simulink model "NewMODEL"  (R2023a)
settings: Solver=VariableStepAuto  StartTime=0.0  StopTime=6  RelTol=1e-3
values from neighbouring files (symbols this model uses):
  A_lift = 3    [Main.m]    (also in SweepTest.m; myActiveSuspensions.mat)
  AO = A-KO*C    [Main.m]    (also in SweepTest.m; myActiveSuspensions.mat = [-6.29015203402 -9209.07677924 -1030.51480744 -503585.757509)
  Ap = 3.35e-4    (= 0.000335)    [Main.m]    (also in SweepTest.m; myActiveSuspensions.mat)
  BO = B1-KO*D1    [Main.m]    (also in SweepTest.m; myActiveSuspensions.mat = [0 0 0 0 154.5])
  Cd_lift = 0.5    [Main.m]    (also in SweepTest.m; myActiveSuspensions.mat)
  Ceps = [1 0 0 0 0 0 ... (first row only)    [Main.m]    (also in SweepTest.m; myActiveSuspensions.mat = [1 0 0 0 0 0 -98.3050847458 1 0 1 0 0 ... (48 elements, 8x6))
  D1eps = [0; 0; 0; 0; 0; 0; 0; 0]    [Main.m]    (also in SweepTest.m; myActiveSuspensions.mat = [0 0 0 0 0 0 0 0])
  DT = 1e-4    (= 0.0001)    [Main.m]    (also in SweepTest.m; myActiveSuspensions.mat)
  e0 = y0(1) - r0    [Main.m]    (also in SweepTest.m; myActiveSuspensions.mat = 0)
  KI = K(:,n+1:n+m)    [Main.m]    (also in SweepTest.m; myActiveSuspensions.mat = -0.35355339059)
  KO = Km.'    [Main.m]    (also in SweepTest.m; myActiveSuspensions.mat = [0.176588896426 58.0307081185 2.94746555023 -226.466108515 -)
  KS = K(:,1:n)    [Main.m]    (also in SweepTest.m; myActiveSuspensions.mat = [3465.7518789 327.330365312 55.983697187 9.36087983472 -400.)
  mi = 1e-7    (= 1e-07)    [Main.m]    (also in SweepTest.m; myActiveSuspensions.mat)
  myVars = rmfield(myVars, "kerO")    [Main.m]    (also in SweepTest.m = rmfield(myVars, "mdl"))
  n = size(V)    [JCF.m]    (also in Main.m = 5; SweepTest.m = 5; myActiveSuspensions.mat = 5)
  p = 1    [Main.m]    (also in SweepTest.m; myActiveSuspensions.mat)
  q = length(index{i})    [JCF.m]    (also in Main.m = 3; SweepTest.m = 3; myActiveSuspensions.mat = 3)
  r0 = - g*ms/ks + l0s + Lift/ks    (= 0.597040517241)    [Main.m]    (also in SweepTest.m; myActiveSuspensions.mat)
  rho_lift = 1.225    [Main.m]    (also in SweepTest.m; myActiveSuspensions.mat)
  v = 10    [Main.m]    (also in SweepTest.m; myActiveSuspensions.mat)
  w0 = [d0; nu0; r0]    [Main.m]    (also in SweepTest.m; myActiveSuspensions.mat = [0 -91.875 0 0 0 0.597040517241])
  x0 = [- g*ms/ks + l0s + Lift/ks ... (first row only)    [Main.m]    (also in SweepTest.m; myActiveSuspensions.mat = [0.597040517241 0 0.3385371843 0 0])
  x_init = [(- g*ms/ks + l0s + Lift/ks) - Diseq ... (first row only)    [Main.m]    (also in SweepTest.m; myActiveSuspensions.mat = [0.597040517241 0 0.3385371843 0 0])
  x_tilde_init = x_init - x0    [Main.m]    (also in SweepTest.m; myActiveSuspensions.mat = [0 0 0 0 0])
  XOinit = x_tilde_init    [Main.m]    (also in SweepTest.m; myActiveSuspensions.mat = [0 0 0 0 0])
  y0 = [x0(1) ... (first row only)    [Main.m]    (also in SweepTest.m; myActiveSuspensions.mat = [0.597040517241 0.935577701542 6.16606577473e-15])
libraries: simulink x3
settings Model: Creator=aleze  LastModifiedBy=aleze

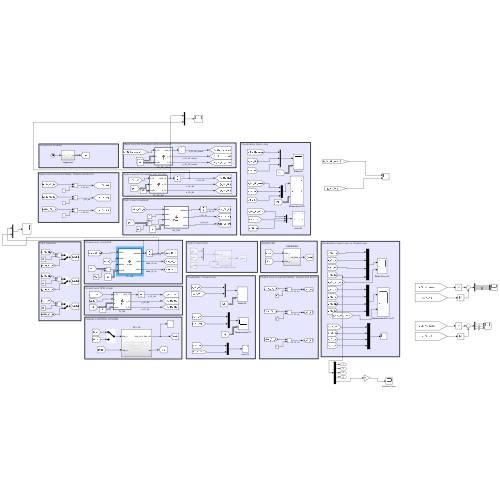
[thumbnail: Simulink's stored preview of the top-level diagram]
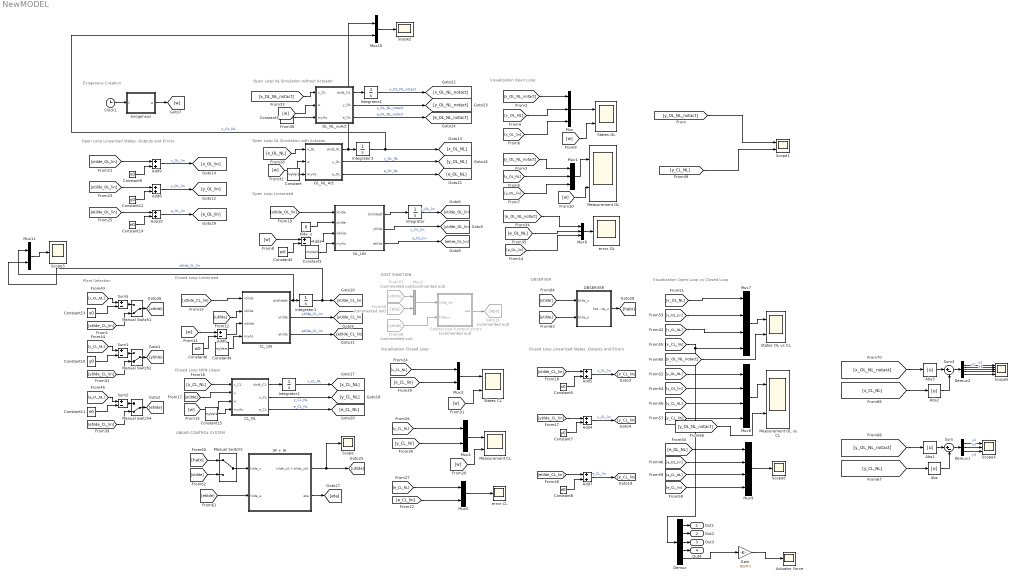
== system NewMODEL ==
  note: Closed Loop Linearized
  note: Open Loop NL Simulation without Actuator
  note: Closed Loop NON Linear
  note: Open Loop Linearized
  note: Exogenous Creation
  note: LINEAR CONTROL SYSTEM
  note: Visualization Open Loop
  note: OBSERVER
  note: Visualization Closed Loop
  note: Open Loop Linearized States, Outputs and Errors
  note: Visualization Open Loop vs Closed Loop
  note: Plant Selection
  note: Closed Loop Linearized States, Outputs and Errors
  note: Open Loop NL Simulation with Actuator
  note: COST FUNCTION
  Abs{,1..3} (4 alike) : Abs  SaturateOnIntegerOverflow=off
  Actuator Force : Scope
  Add{4..5,7..10} (6 alike) : Sum
  Add2 : Sum  Inputs=+-
  Add6 : Sum  Inputs=+-
  CL_LIN : MATLAB Function  TreatAsAtomicUnit=on
  CL_NL : MATLAB Function  TreatAsAtomicUnit=on
  Clock1 : Clock
  Constant{,1,3..4,15} (5 alike) : Constant  Value=myVars  OutDataTypeStr=Bus: slBus1
  Constant10 : Constant  Value=y0
  Constant11 : Constant  Value=e0
  Constant12 : Constant  Value=y0
  Constant13 : Constant  Value=x0
  Constant14 : Constant  Value=e0
  Constant2 : Constant  Value=w0
  Constant5 : Constant  Value=x0
  Constant6 : Constant  Value=w0
  Constant7 : Constant  Value=y0
  Constant8 : Constant  Value=e0
  Constant9 : Constant  Value=x0
  Control cost function errors : Subsystem  Commented=on
  Demux : Demux  Outputs=5
  Demux1 : Demux  Outputs=3
  Demux2 : Demux  Outputs=5
  From37 : From  Commented=on  GotoTag=xtilde
  From38 : From  Commented=on  GotoTag=utilde
  From40 : From  Commented=on  GotoTag=eta
  Gain : Gain  Gain=Ap/mi
  Goto15 : Goto  Commented=on  GotoTag=eps
  Integrator : Integrator  InitialCondition=x_tilde_init
  Integrator1 : Integrator  InitialCondition=x_tilde_init
  Integrator2 : Integrator  InitialCondition=x_init
  Integrator3 : Integrator  InitialCondition=x_init
  Integrator4 : Integrator  InitialCondition=x_init
  Manual Switch1 : ManualSwitch  CurrentSetting=0
  Manual Switch2 : ManualSwitch  CurrentSetting=0
  Manual Switch4 : ManualSwitch  CurrentSetting=0
  Manual Switch5 : ManualSwitch
  Measurement CL : Scope  NumInputPorts=2
  Measurement OL : Scope  NumInputPorts=2
  Measurement OL vs CL : Scope  NumInputPorts=2
  Mux : Mux  Inputs=3
  Mux1 : Mux  Inputs=3
  Mux{3..5,10..11} (5 alike) : Mux  Inputs=2
  Mux2 : Mux  Commented=on  Inputs=2
  Mux6 : Mux  Inputs=3
  Mux7 : Mux
  Mux8 : Mux
  Mux9 : Mux
  OBSERVER : Subsystem
  OL_LIN : MATLAB Function  TreatAsAtomicUnit=on
  OL_NL_Act : MATLAB Function  TreatAsAtomicUnit=on
  OL_NL_noAct : MATLAB Function  TreatAsAtomicUnit=on
  SF + IA : Subsystem
  Scope{,2..3,6} (4 alike) : Scope
  Scope1 : Scope  NumInputPorts=2
  Scope4 : Scope  NumInputPorts=3
  Scope5 : Scope  NumInputPorts=5
  States CL : Scope  NumInputPorts=2
  States OL : Scope  NumInputPorts=2
  States OL vs CL : Scope  NumInputPorts=2
  Sum : Sum  Inputs=|+-
  Sum1 : Sum  Inputs=+-
  Sum2 : Sum  Inputs=+-
  Sum3 : Sum  Inputs=|+-
  Sum5 : Sum  Inputs=+-
  error CL : Scope
  error OL : Scope
  exogenous : Subsystem
  tilde_u : Constant  Value=0  VectorParams1D=off
  Out1 : Outport
  Out2 : Outport  Port=2
  Out3 : Outport  Port=3
  Out4 : Outport  Port=4
  wires:
  [xtilde_CL_lin] -> CL_LIN/1(xtilde)
  [x_OL_NL] -> OL_NL_Act/1(x_OL)
  Sum5/1 -> Manual Switch1/1
  [xtilde_CL_lin] -> Manual Switch1/2
  Mux6/1 -> error OL/1
  Add7/1 -> [e_CL_lin]  "e_CL_lin"
  Add5/1 -> [x_CL_lin]  "x_CL_lin"
  Demux1/3 -> Scope4/3  "y3"
  [x_OL_NL_notact] -> OL_NL_noAct/1(x_OL)
  Integrator2/1 -> [x_CL_NL]  "x_CL_NL"
  Constant10/1 -> Sum1/2
  [x_CL_NL] -> Abs2/1
  [utilde] -> CL_LIN/2(utilde)
  OL_NL_Act/3(e_OL) -> [e_OL_NL]  "e_OL_NL"
  Constant6/1 -> Add6/2
  [w] -> Add6/1
  [x_CL_lin] -> Mux3/2
  Sum2/1 -> Manual Switch4/1
  [x_CL_NL] -> Mux7/3
  [w] -> States OL/2
  [y_OL_NL_notact] -> Scope1/1
  OL_LIN/1(dxtildedt) -> Integrator/1
  Clock1/1 -> exogenous/1(t)
  [ytilde_CL_lin] -> Manual Switch2/2
  Integrator1/1 -> Mux11/2, [xtilde_CL_lin]  "xtilde_CL_lin"
  CL_NL/2(y_CL) -> [y_CL_NL]  "y_CL_NL"
  OL_NL_noAct/3(e_OL) -> [e_OL_NL_notact]  "e_OL_NL_notact"
  [w] -> Measurement CL/2
  [x_OL_NL] -> Mux7/1
  Manual Switch1/1 -> [xtilde]
  [y_CL_NL] -> Sum1/1
  OL_NL_Act/2(y_OL) -> [y_OL_NL]  "y_OL_NL"
  Manual Switch4/1 -> [etilde]
  [w] -> States CL/2
  Constant5/1 -> Add5/2
  [e_CL_NL] -> Mux9/3
  [x_OL_NL] -> Mux/2
  OL_NL_Act/1(dxdt_OL) -> Mux10/1, Integrator3/1
  [y_OL_NL] -> Mux1/2
  Control cost function errors/1(eps) -> Goto15/1
  Add2/1 -> OL_LIN/3(wtilde)
  Mux1/1 -> Measurement OL/1
  CL_NL/3(e_CL) -> [e_CL_NL]  "e_CL_NL"
  exogenous/1(w) -> [w]
  [x_CL_lin] -> Demux/1, Mux7/4
  Mux4/1 -> Measurement CL/1
  OL_NL_noAct/1(dxdt_OL) -> Integrator4/1
  Constant11/1 -> Sum2/2
  [w] -> Measurement OL/2
  Sum/1 -> Demux1/1
  [e_OL_NL] -> Mux6/2
  [e_OL_lin] -> Mux6/3
  CL_LIN/2(ytilde) -> [ytilde_CL_lin]  "ytilde_CL_lin"
  [etilde_OL_lin] -> Add10/1
  CL_LIN/1(dxtildedt) -> Mux11/1, Integrator1/1
  Abs/1 -> Sum/2
  Demux/2 -> Out2/1
  Demux/5 -> Gain/1
  Mux/1 -> States OL/1
  Mux11/1 -> Scope3/1
  [ytilde] -> OBSERVER/2(tilde_y)
  Demux1/2 -> Scope4/2  "y2"
  Gain/1 -> Actuator Force/1
  Mux10/1 -> Scope2/1
  From37/1 -> Mux2/1
  Demux2/3 -> Scope5/3  "y3"
  Demux2/1 -> Scope5/1  "y1"
  Add9/1 -> [x_OL_lin]  "x_OL_lin"
  [etilde_CL_lin] -> Manual Switch4/2
  Demux1/1 -> Scope4/1  "y1"
  Demux2/2 -> Scope5/2  "y2"
  Mux8/1 -> Measurement OL vs CL/1
  [w] -> OL_NL_Act/2(w)
  [y_CL_NL] -> Mux8/3
  [e_CL_lin] -> Mux5/2
  Abs2/1 -> Sum3/2
  Integrator/1 -> [xtilde_OL_lin]  "x_OL_lin"
  [x_CL_NL] -> CL_NL/1(x_CL)
  Mux5/1 -> error CL/1
  Mux9/1 -> Scope6/1
  Add10/1 -> [e_OL_lin]  "e_OL_lin"
  [x_OL_lin] -> Mux7/2
  [w] -> Add2/1
  Constant12/1 -> Add8/2
  [e_CL_lin] -> Mux9/4
  Sum1/1 -> Manual Switch2/1
  [ytilde_OL_lin] -> Add8/1
  CL_NL/1(dxdt_CL) -> Integrator2/1
  Mux3/1 -> States CL/1
  Constant14/1 -> Add10/2
  [e_CL_NL] -> Mux5/1
  [y_OL_NL] -> Mux8/1
  Mux7/1 -> States OL vs CL/1
  [e_OL_NL] -> Mux9/1
  [y_OL_lin] -> Mux8/2
  SF + IA/2(eta) -> [eta]
  Demux2/5 -> Scope5/5
  Abs1/1 -> Sum/1
  [x_OL_NL_notact] -> Mux/1
  OL_LIN/2(ytilde) -> [ytilde_OL_lin]  "y_OL_lin"
  [w] -> OL_NL_noAct/2(w)
  [utilde] -> CL_NL/2(u)
  Constant13/1 -> Sum5/2
  Mux2/1 -> Control cost function errors/1(tilde_xe)
  [y_OL_NL_notact] -> Abs1/1
  Constant/1 -> OL_NL_Act/3(myAs)
  [e_CL_NL] -> Sum2/1
  [utilde] -> OBSERVER/1(tilde_u)
  [y_CL_lin] -> Mux8/4
  Constant1/1 -> OL_LIN/4(myAs)
  Constant7/1 -> Add4/2
  Constant3/1 -> OL_NL_noAct/3(myAs)
  [w] -> CL_NL/3(w)
  Constant15/1 -> CL_NL/4(myAs)
  [y_CL_lin] -> Mux4/2
  Constant4/1 -> CL_LIN/4(myAs)
  [hatx] -> Manual Switch5/1
  [xtilde_OL_lin] -> OL_LIN/1(xtilde)
  Constant8/1 -> Add7/2
  Demux/4 -> Out4/1
  OL_LIN/3(etilde) -> [etilde_OL_lin]  "e_OL_lin"
  [x_CL_NL] -> Sum5/1
  Manual Switch5/1 -> SF + IA/1(tilde_x)
  [ytilde_CL_lin] -> Add4/1
  tilde_u/1 -> OL_LIN/2(utilde)
  [x_OL_NL_notact] -> Abs3/1
  [y_OL_NL_notact] -> Mux1/1
  [y_CL_NL] -> Scope1/2
  Add6/1 -> CL_LIN/3(wtilde)
  [etilde_CL_lin] -> Add7/1
  Demux/1 -> Out1/1
  From38/1 -> Control cost function errors/2(tilde_u)
  Demux2/4 -> Scope5/4
  Constant2/1 -> Add2/2
  SF + IA/1(tilde_uS + tilde_uIA) -> [utilde], Scope/1
  Abs3/1 -> Sum3/1
  [y_CL_NL] -> Mux4/1
  Integrator3/1 -> Mux10/2, [x_OL_NL]  "x_OL_NL"
  Manual Switch2/1 -> [ytilde]
  [e_OL_NL_notact] -> Mux6/1
  [xtilde_CL_lin] -> Add5/1
  [xtilde] -> Manual Switch5/2
  OBSERVER/1(hat_tilde_x) -> [hatx]
  Add4/1 -> [y_CL_lin]  "y_CL_lin"
  [y_OL_NL_notact] -> Measurement OL vs CL/2
  CL_LIN/3(etilde) -> [etilde_CL_lin]  "etilde_CL_lin"
  Demux/3 -> Out3/1
  [etilde] -> SF + IA/2(tilde_e)
  [e_OL_lin] -> Mux9/2
  [y_OL_lin] -> Mux1/3
  [x_CL_NL] -> Mux3/1
  Integrator4/1 -> [x_OL_NL_notact]  "x_OL_NL_notact"
  [x_OL_NL_notact] -> States OL vs CL/2
  [y_CL_NL] -> Abs/1
  From40/1 -> Mux2/2
  OL_NL_noAct/2(y_OL) -> [y_OL_NL_notact]  "y_OL_NL_notact"
  [xtilde_OL_lin] -> Add9/1
  Constant9/1 -> Add9/2
  Add8/1 -> [y_OL_lin]  "y_OL_lin"
  [x_OL_lin] -> Mux/3
  Sum3/1 -> Demux2/1

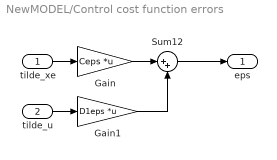
== system NewMODEL/Control cost function errors ==
  tilde_xe : Inport
  tilde_u : Inport  Port=2
  Gain : Gain  Gain=Ceps  Multiplication=Matrix(K*u)
  Gain1 : Gain  Gain=D1eps  Multiplication=Matrix(K*u)
  Sum12 : Sum  Inputs=|++
  eps : Outport
  wires:
  Gain1/1 -> Sum12/2
  Gain/1 -> Sum12/1
  Sum12/1 -> eps/1
  tilde_xe/1 -> Gain/1
  tilde_u/1 -> Gain1/1

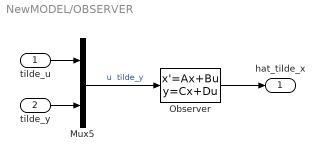
== system NewMODEL/OBSERVER ==
  tilde_u : Inport
  tilde_y : Inport  Port=2
  Mux5 : Mux  Inputs=2
  Observer : StateSpace  A=AO  B=[BO KO]  C=eye(n)  D=zeros(n, p+q)  InitialCondition=XOinit  ParameterTunability=Unconstrained
  hat_tilde_x : Outport
  wires:
  tilde_u/1 -> Mux5/1
  tilde_y/1 -> Mux5/2
  Mux5/1 -> Observer/1  "u  tilde_y"
  Observer/1 -> hat_tilde_x/1

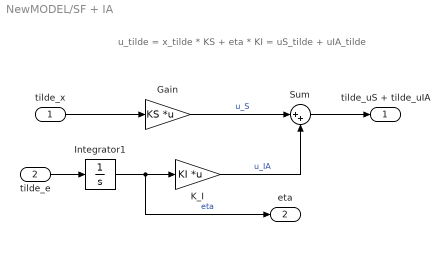
== system NewMODEL/SF + IA ==
  note: u_tilde = x_tilde * KS + eta * KI = uS_tilde + uIA_tilde
  tilde_x : Inport
  tilde_e : Inport  Port=2
  Gain : Gain  Gain=KS  Multiplication=Matrix(K*u)
  Integrator1 : Integrator
  K_I : Gain  Gain=KI  Multiplication=Matrix(K*u)
  Sum : Sum  Inputs=|++
  tilde_uS + tilde_uIA : Outport
  eta : Outport  Port=2
  wires:
  Integrator1/1 -> eta/1, K_I/1  "eta"
  tilde_e/1 -> Integrator1/1
  tilde_x/1 -> Gain/1
  K_I/1 -> Sum/2  "u_IA"
  Sum/1 -> tilde_uS + tilde_uIA/1
  Gain/1 -> Sum/1  "u_S"

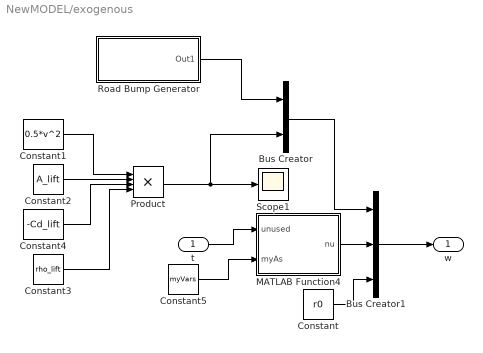
== system NewMODEL/exogenous ==
  t : Inport
  Bus Creator : BusCreator  Inputs=2
  Bus Creator1 : BusCreator  Inputs=3
  Constant : Constant  Value=r0
  Constant1 : Constant  Value=0.5*v^2  SampleTime=DT
  Constant2 : Constant  Value=A_lift  SampleTime=DT
  Constant3 : Constant  Value=rho_lift  SampleTime=DT
  Constant4 : Constant  Value=-Cd_lift  SampleTime=DT
  Constant5 : Constant  Value=myVars  OutDataTypeStr=Bus: slBus1
  MATLAB Function4 : MATLAB Function  TreatAsAtomicUnit=on  SystemSampleTime=DT
  Product : Product  Inputs=4
  Road Bump Generator : Subsystem
  Scope1 : Scope
  w : Outport
  wires:
  Constant1/1 -> Product/1
  Road Bump Generator/1(Out1) -> Bus Creator/1
  Constant2/1 -> Product/2
  t/1 -> MATLAB Function4/1(unused)
  Constant3/1 -> Product/4
  Constant4/1 -> Product/3
  Product/1 -> Bus Creator/2, Scope1/1
  Bus Creator/1 -> Bus Creator1/1
  MATLAB Function4/1(nu) -> Bus Creator1/2
  Constant/1 -> Bus Creator1/3
  Bus Creator1/1 -> w/1
  Constant5/1 -> MATLAB Function4/2(myAs)

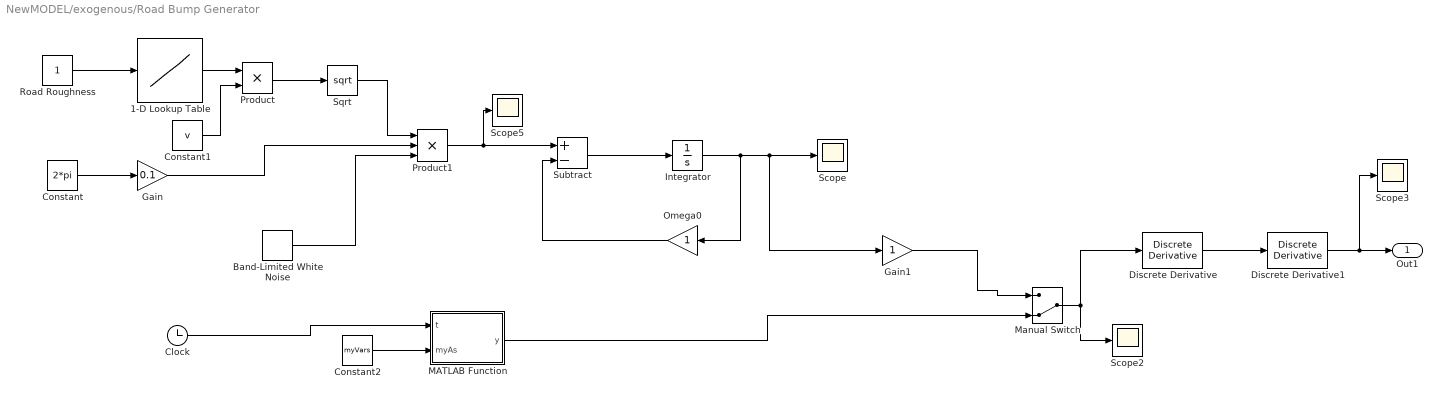
== system NewMODEL/exogenous/Road Bump Generator ==
  1-D Lookup Table : Lookup_n-D  NumberOfTableDimensions=1  BreakpointsForDimension1=[1;2;3;4;5;6;7;8]  Table=[1.6e-05;6.4e-05;0.000256;0.001024;0.004096;0.016384;0.065536;0.262144]  InternalRulePriority=Speed  RndMeth=Simplest
  Band-Limited White Noise : simulink/Sources/Band-Limited White Noise  Cov=0.1  Ts=0.01  seed=[23341]
  Clock : Clock
  Constant : Constant  Value=2*pi
  Constant1 : Constant  Value=v
  Constant2 : Constant  Value=myVars  OutDataTypeStr=Bus: slBus1
  Discrete Derivative : simulink/Quick Insert/Discrete/Discrete Derivative  gainval=1.0  ICPrevScaledInput=0.0  OutMin=[]  OutMax=[]  OutDataType=fixdt(1, 16)  OutScaling=2^-10  DoSatur=off
  Discrete Derivative1 : simulink/Quick Insert/Discrete/Discrete Derivative  gainval=1.0  ICPrevScaledInput=0.0  OutMin=[]  OutMax=[]  OutDataType=fixdt(1, 16)  OutScaling=2^-10  DoSatur=off
  Gain : Gain  Gain=0.1
  Gain1 : Gain
  Integrator : Integrator
  MATLAB Function : MATLAB Function  TreatAsAtomicUnit=on
  Manual Switch : ManualSwitch  CurrentSetting=0
  Omega0 : Gain
  Product : Product
  Product1 : Product  Inputs=3
  Road Roughness : Constant
  Scope{,2..3,5} (4 alike) : Scope
  Sqrt : Sqrt
  Subtract : Sum  Inputs=+-
  Out1 : Outport
  wires:
  Subtract/1 -> Integrator/1
  Road Roughness/1 -> 1-D Lookup Table/1
  Clock/1 -> MATLAB Function/1(t)
  1-D Lookup Table/1 -> Product/1
  Sqrt/1 -> Product1/1
  Constant/1 -> Gain/1
  Band-Limited White Noise/1 -> Product1/3
  Omega0/1 -> Subtract/2
  MATLAB Function/1(y) -> Manual Switch/2
  Product1/1 -> Scope5/1, Subtract/1
  Integrator/1 -> Omega0/1, Gain1/1, Scope/1
  Constant1/1 -> Product/2
  Product/1 -> Sqrt/1
  Gain/1 -> Product1/2
  Gain1/1 -> Manual Switch/1
  Discrete Derivative/1 -> Discrete Derivative1/1
  Discrete Derivative1/1 -> Out1/1, Scope3/1
  Manual Switch/1 -> Scope2/1, Discrete Derivative/1
  Constant2/1 -> MATLAB Function/2(myAs)

== matlab function NewMODEL/CL_LIN ==
  data: xtilde input; utilde input; dxtildedt output; wtilde input; ytilde output; etilde output; myAs input
function [dxtildedt, ytilde, etilde] = Plant(xtilde,utilde,wtilde,myAs)

%% Plant Parameters
ks = myAs.ks; % [N/m] spring coefficient
kt = myAs.kt; % [N/m] tyre elastic coefficient
mu = myAs.mu;
ms = myAs.ms;
g = myAs.g;
betas = myAs.betas; % damping coefficient 

A_lift = 3;
Cd_lift = 0.5; 
rho_lift = 1.225; %kg/m^3
v = 10; %[m/s] speed of the car
Lift = 0.5*A_lift*Cd_lift*(v^2)*rho_lift;           % da A_lift fino a qua levo?

%% ACTUATOR PARAMETERS
beta = myAs.beta; %1/sec
mi = myAs.mi; % scale coefficient to improve numerical conditioning of P
gamma = myAs.gamma; % N/m^(5/2)kg^(1/2)
Ap = myAs.Ap; % m^2
alfa = myAs.alfa; % N/m^5

%% LINEARIZED MATRIXES

N = (ms+mu)/(ms*mu);

A = myAs.A;

B1 = myAs.B1;

B2 = myAs.B2;

C = myAs.C;

D1 = myAs.D1;

D2 = myAs.D2;

Ce = myAs.Ce;  

De1 = myAs.De1;

De2 = myAs.De2;

dxtildedt = A*xtilde+B1*utilde+B2*wtilde;
ytilde = C*xtilde+D1*utilde+D2*wtilde;
etilde = Ce*xtilde+De1*utilde+De2*wtilde;

== matlab function NewMODEL/OL_LIN ==
  data: xtilde input; utilde input; dxtildedt output; wtilde input; ytilde output; etilde output; myAs input
function [dxtildedt, ytilde, etilde] = Plant(xtilde,utilde,wtilde,myAs)

%% Plant Parameters
ks = myAs.ks; % [N/m] spring coefficient
kt = myAs.kt; % [N/m] tyre elastic coefficient
mu = myAs.mu;
ms = myAs.ms;
g = myAs.g;
betas = myAs.betas; % damping coefficient 

A_lift = myAs.A_lift;
Cd_lift = myAs.Cd_lift; 
rho_lift = myAs.rho_lift; %kg/m^3
v = myAs.v; %[m/s] speed of the car
Lift = 0.5*A_lift*Cd_lift*(v^2)*rho_lift;           %Forse da A_lift a qua non serve

%% ACTUATOR PARAMETERS
beta = myAs.beta; %1/sec
mi = myAs.mi; % scale coefficient to improve numerical conditioning of P
gamma = myAs.gamma; % N/m^(5/2)kg^(1/2)
Ap = myAs.Ap; % m^2
alfa = myAs.alfa; % N/m^5

%% LINEARIZED MATRIXES

N = (ms+mu)/(ms*mu);

A = myAs.A;

B1 = myAs.B1;

B2 = myAs.B2;

C = myAs.C;

D1 = myAs.D1;

D2 = myAs.D2;

Ce = myAs.Ce;  

De1 = myAs.De1;

De2 = myAs.De2;

dxtildedt = A*xtilde+B1*utilde+B2*wtilde;
ytilde = C*xtilde+D1*utilde+D2*wtilde;
etilde = Ce*xtilde+De1*utilde+De2*wtilde;

== matlab function NewMODEL/OL_NL_Act ==
  data: dxdt_OL output; x_OL input; y_OL output; w input; e_OL output; myAs input
function [dxdt_OL, y_OL, e_OL] = f(x_OL, w,myAs)

x1 = x_OL(1);
x2 = x_OL(2);
x3 = x_OL(3);
x4 = x_OL(4);
x5 = x_OL(5);

% Disturbance
d = w(1);
Lift = w(2);

% Noise
ni1 = w(3);
ni2 = w(4);
ni3 = w(5);

% Reference
r0 = w(6);


%% Plant Parameters
ks = myAs.ks; % [N/m] spring coefficient
mu = myAs.mu;
ms = myAs.ms;
l0s = myAs.l0s; % [m] lenght of the sprung for which the force is 0
g = myAs.g;
betas = myAs.betas; % damping coefficient 

%% ACTUATOR PARAMETERS
beta = myAs.beta; %1/sec
mi = myAs.mi; % scale coefficient to improve numerical conditioning of P
Ap = myAs.Ap; % m^2
alfa = myAs.alfa; % N/m^5

%% State Space Model

N = (mu+ms)/(ms*mu); 

dxdt1 = x2;
dxdt2 = N*(-ks*(x1-l0s)-betas*x2) - 1/mu*(ft(x3,myAs)) + Lift/ms + N*(Ap/mi)*x5;
dxdt3 = x4;
dxdt4 = -g + ks/mu*(x1-l0s) + betas/mu*x2 + 1/mu*(ft(x3,myAs)) - 1/mu*(Ap/mi)*x5 - d;
dxdt5 = -beta*x5 - mi*alfa*Ap*x2; % + mi*gamma*u;

dxdt_OL = [dxdt1;dxdt2;dxdt3;dxdt4;dxdt5];

y_OL = [x1 + ni1 
     x1 + x3 + ni2 
     1/ms*(Lift-ms*g-ks*(x1-l0s) - betas*x2 + x5*Ap/mi) + ni3];

e_OL = x1 + ni1 - r0;

end


%% SUPPORT FUNCTIONS

function f = ft(s,myAs)
l0t = myAs.l0t; % [m]
kt = myAs.kt; %tyre elastic coefficient
if s > l0t
    f = 0;
    dxdt3 = 0;                      % ???
else
    f = -kt*(s-l0t);
end
end

== matlab function NewMODEL/exogenous/MATLAB Function4 ==
  data: unused input; nu output; myAs input
function nu = noises(~, myAs)

%% Noises Function
std_pot = myAs.std_pot; % [m] potentiomenter standard deviation
std_laser = myAs.std_laser; %standard deviation laser
std_acc = myAs.std_acc; % [m/s^2] accelerometer standard deviation
nu = [std_pot*(2*rand(1)-1)
      std_laser*(2*rand(1)-1)
      std_acc*(2*rand(1)-1)];

end

== matlab function NewMODEL/exogenous/Road Bump Generator/MATLAB Function ==
  data: t input; y output; myAs input
function y = fcn(t, myAs)

%% Parameters definition

v = myAs.v; % [m/s] speed of the vehicle

p = v*t; % [m] position that varies with time

pg = 20; % [m] pg is the position of the BEGINNING of the bump

l = 10; % [m] lenght of the hole/bump
h = 0.10; % [m] thickness of the hole/bump

lmat = [l^4 l^5 l^6 l^7 l^8; (l/2)^4 (l/2)^5 (l/2)^6 (l/2)^7 (l/2)^8; 4*l^3 5*l^4 6*l^5 7*l^6 8*l^7; 12*l^2 20*l^3 30*l^4 42*l^5 56*l^6; 24*l 60*l^2 120*l^3 210*l^4 336*l^5;];
lmatinv = inv(lmat);

cmat = zeros(5,1);
hmat = [0 h 0 0 0]';

cmat = lmatinv * hmat;

% Road profile function

if (p>pg && p-pg < l)
    sum = 0;
    for i = 0:8
        if i > 3
            sum = sum + cmat(i-3)*(p-pg)^(i);
        end
    end
    y = sum;
else
    y = 0;
end

== matlab function NewMODEL/CL_NL ==
  data: dxdt_CL output; x_CL input; u input; y_CL output; w input; e_CL output; myAs input
function [dxdt_CL, y_CL, e_CL] = f(x_CL, u, w,myAs)

x1 = x_CL(1);
x2 = x_CL(2);
x3 = x_CL(3);
x4 = x_CL(4);
x5 = x_CL(5);

% Disturbance
d = w(1);
Lift = w(2);

% Noise
ni1 = w(3);
ni2 = w(4);
ni3 = w(5);

% Reference
r0 = w(6);


%% Plant Parameters
ks = myAs.ks; % [N/m] spring coefficient
mu = myAs.mu;
ms = myAs.ms;
l0s = myAs.l0s; % [m] lenght of the sprung for which the force is 0
g = myAs.g;
betas = myAs.betas; % damping coefficient 

%% ACTUATOR PARAMETERS
beta = myAs.beta; %1/sec
mi = myAs.mi; % scale coefficient to improve numerical conditioning of P
gamma = myAs.gamma; % N/m^(5/2)kg^(1/2)
Ap = myAs.Ap; % m^2
alfa = myAs.alfa; % N/m^5

%% State Space Model

N = (mu+ms)/(ms*mu); 

dxdt1 = x2;
dxdt2 = N*(-ks*(x1-l0s)-betas*x2) - 1/mu*(ft(x3,myAs)) + Lift/ms + N*(Ap/mi)*x5;
dxdt3 = x4;
dxdt4 = -g + ks/mu*(x1-l0s) + betas/mu*x2 + 1/mu*(ft(x3,myAs)) - 1/mu*(Ap/mi)*x5 - d;
dxdt5 = -beta*x5 - mi*alfa*Ap*x2 + mi*gamma*u;

dxdt_CL = [dxdt1;dxdt2;dxdt3;dxdt4;dxdt5];

y_CL = [x1 + ni1 
     x1 + x3 + ni2 
     1/ms*(Lift-ms*g-ks*(x1-l0s) - betas*x2 + x5*Ap/mi) + ni3];

e_CL = x1 + ni1 - r0;

end


%% SUPPORT FUNCTIONS

function f = ft(s,myAs)

l0t = myAs.l0t; % [m]
kt = myAs.kt; %tyre elastic coefficient
if s > l0t
    f = 0;
else
    f = -kt*(s-l0t);
end
end

== matlab function NewMODEL/OL_NL_noAct ==
  data: dxdt_OL output; x_OL input; y_OL output; w input; e_OL output; myAs input
function [dxdt_OL, y_OL, e_OL] = f(x_OL,w, myAs)

x1 = x_OL(1);
x2 = x_OL(2);
x3 = x_OL(3);
x4 = x_OL(4);

% Disturbance
d=w(1);
Lift = w(2);

% Noise
ni1 = w(3);
ni2 = w(4);
ni3 = w(5);

% Reference
r0 = w(6);

%% Plant Parameters
ks = myAs.ks; % [N/m] spring coefficient
mu = myAs.mu;
ms = myAs.ms;
l0s = myAs.l0s; % [m] lenght of the sprung for which the force is 0
g = myAs.g;
betas = myAs.betas; % damping coefficient 

%% STATE DYNAMICS

N = (mu+ms)/(ms*mu); 

dxdt_OL = [x2
    N*(-ks*(x1-l0s)-betas*x2) - 1/mu*ft(x3,myAs) + Lift/ms
    x4
    -g + ks/mu*(x1-l0s) + betas/mu*x2 + 1/mu*ft(x3,myAs) - d
    0];

y_OL = [x1 + ni1 
     x1 + x3 + ni2 
     1/ms*(Lift-ms*g-ks*(x1-l0s) - betas*x2) + ni3];

e_OL = x1 + ni1 - r0;

end


%% SUPPORT FUNCTIONS

function f = ft(s, myAs)
l0t = myAs.l0t; % [m]
kt = myAs.kt; %tyre elastic coefficient
if s > l0t
    f = 0;
else
    f = -kt*(s-l0t);
end
end
